simulink model "wasserpumpe"  (R2016b)
settings: Solver=VariableStepAuto  StartTime=0.0  StopTime=10  MaxStep=0.05  RelTol=1e-3  EnableMultiTasking=on
libraries: sh_lib x9, fl_lib x7, nesl_utility x4
CloseFcn:
  | try,close(h1_sh_well_jet_pump),end
  | clear h1_sh_well_jet_pump
  | 
  | 
  | clear simlog_sh_well_jet_pump
Description:
  | Well with Jet Pump
  | 
  | Copyright 2008-2016 The MathWorks, Inc.
settings Model: ExtModeAutoUpdateStatusClock=off  Creator=MathWorks  LastModifiedBy=user
settings DataIOCC: LimitDataPoints=on  MaxDataPoints=10000  SaveFormat=Array  SignalLoggingSaveFormat=ModelDataLogs  SignalLoggingName=logsout_sh_well_jet_pump
settings OptimizationCC: ExpressionDepthLimit=2147483647  InitFltsAndDblsToZero=on  LifeSpan=inf
settings DebuggingCC: SaveWithParameterizedLinksMsg=none  UnderspecifiedInitializationDetection=Classic  MergeDetectMultiDrivingBlocksExec=none  SignalResolutionControl=TryResolveAllWithWarning  SolverPrmCheckMsg=warning  MultiTaskDSMMsg=warning  MultiTaskCondExecSysMsg=none  FcnCallInpInsideContextMsg=warning  AllowSymbolicDim=off  StateNameClashWarn=warning  SFUnexpectedBacktrackingDiag=warning  SFNoUnconditionalDefaultTransitionDiag=warning  SFExecutionAtInitializationDiag=none
settings HardwareCC: ProdBitPerPointer=32  ProdBitPerSizeT=32  ProdBitPerPtrDiffT=32  ProdLargestAtomicFloat=None  ProdIntDivRoundTo=Undefined  ProdEndianess=Unspecified  ProdWordSize=32  ProdHWDeviceType=32-bit Generic
settings ModelReferenceCC: PropagateSignalLabelsOutOfModel=off
settings GRTTargetCC: TargetFcnLib=ansi_tfl_tmw.mat  TargetLangStandard=C89/C90 (ANSI)  GeneratePreprocessorConditionals=Disable all  CombineOutputUpdateFcns=off  GRTInterface=on
settings ConfigComp: CovMetricSettings=dw  CovHtmlReporting=on  CovSaveCumulativeToWorkspaceVar=on  CovSaveSingleToWorkspaceVar=on  CovShowResultsExplorer=off  CovExternalEMLEnable=off
settings SimscapeCC: SimscapeLogType=all  SimscapeLogSimulationStatistics=on  SimscapeLogName=simlog_sh_well_jet_pump  SimscapeLogDataHistory=10000

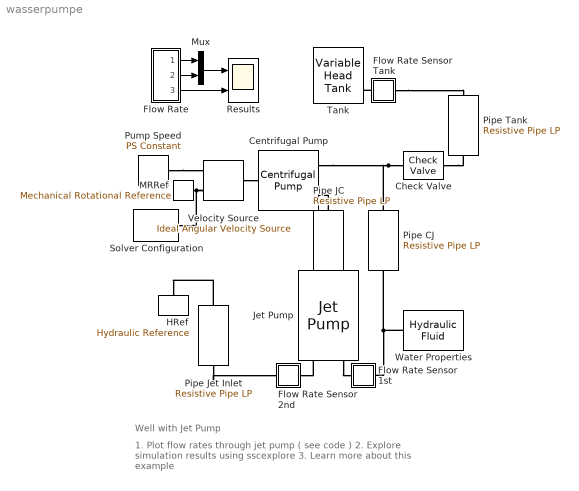
== system wasserpumpe ==
  note: Well with Jet Pump
  note: 1. Plot flow rates through jet pump ( see code )
      | 2. Explore simulation results using sscexplore
      | 3. Learn more about this example
  Centrifugal Pump : sh_lib/Pumps and Motors/Centrifugal Pump  mdl_type=2  c_1=326.8 Pa/(kg/m^3)  c_2=3.104e+4 Pa*s/kg  c_3=1.097e+7 Pa*s^2/(kg*m^3)  c_4=2.136e+5 Pa*s^2/(kg*m^3)  c_f=0.8  design_del=130 lpm  ref_velocity=1.77e+3 rpm  ref_density=940 kg/m^3  leak_resistance=1e+8 Pa/(m^3/s)  T_const=0.1 N*m  trq_press_coeff=1e-6 N*m/Pa  pump_del_1D="[ 0  0.076   0.24   0.35  0.416  0.492] m^3/s"  press_diff_1D=[3.514 3.246 2.6972 2.16 1.627 1.08] bar  pump_del_power_1D="[ 0  0.076   0.24   0.35  0.416  0.492] m^3/s"  power_1D="[0 0.58   1.57  1.79  1.61  1.27] kW"  pump_del_2D=[ 0 50 100 150 200 250 300 350 ] lpm  pump_vel_2D=[ 3.2e+3 3.3e+3 3.4e+3 3.5e+3 ] rpm  press_diff_2D=[ 8.3 8.8 9.3 9.9; 7.8 8.3 8.8 9.4; 7.2 7.6 8.2 8.7; 6.5 7 7.5 8; 5.6 6.1 6.6 7.1; 4.7 5.2 5.7 6.2; 3.4 4 4.4 4.9; 2.3 2.7 3.4 3.6 ] bar  pump_del_power_2D=[ 0 50 100 150 200 250 300 350 ] lpm  power_2D=[ 1.223e+3 1.341e+3 1.467e+3 1.6e+3; 1.414e+3 1.551e+3 1.696e+3 1.85e+3; 1.636e+3 1.794e+3 1.962e+3 2.14e+3; 1.941e+3 2.129e+3 2.326e+3 2.54e+3; 2.224e+3 2.439e+3 2.66e+3 2.91e+3; 2.453e+3 2.691e+3 2.947e+3 3.21e+3; 2.757e+3 3.024e+3 3.307e+3 3.608e+3; 2.945e+3 3.23e+3 3.533e+3 3.854e+3 ] W  interp_method=1  extrap_method=1
  Check Valve : sh_lib/Valves/Directional Valves/Check Valve  area_max=9.65 cm^2  pres_crack=0.055 bar  pres_max=0.172 bar  C_d=0.7  Re_cr=12  A_leak=1e-9 m^2  dynamic=0  tau=0.1 s  area_init=1e-12 m^2
  Flow Rate : Subsystem
  Flow Rate Sensor 1st : Subsystem
      mask Display: disp('Q1');
  Flow Rate Sensor 2nd : Subsystem
      mask Display: disp('Q2');
  Flow Rate Sensor Tank : Subsystem
      mask Display: disp('QT');
  HRef : fl_lib/Hydraulic/Hydraulic Elements/Hydraulic Reference
  Jet Pump : sh_lib/Pumps and Motors/Jet Pump  A_n=3 cm^2  A_th=6 cm^2  a=0.224  K_n=0.05  K_en=0.005  K_th=0.1  K_di=0.14
  MRRef : fl_lib/Mechanical/Rotational Elements/Mechanical Rotational Reference
  Mux : Mux  Inputs=2
  Pipe Jet Inlet : sh_lib/Low-Pressure Blocks/Resistive Pipe LP  cs_type=1  d_in=5 cm  area=1e-4 m^2  D_h=0.0112 m  s_factor=64  length=0.5 m  length_ad=1.5 m  roughness=1.5e-5 m  Re_lam=2e+3  Re_turb=4e+3  elevation_A=0 ft  elevation_B=-0.457 ft
  Pipe Tank : sh_lib/Low-Pressure Blocks/Resistive Pipe LP  cs_type=1  d_in=5 cm  area=1e-4 m^2  D_h=0.0112 m  s_factor=64  length=130 m  length_ad=15.5 m  roughness=1.5e-5 m  Re_lam=2e+3  Re_turb=4e+3  elevation_A=11 m  elevation_B=16 m
  Pipe CJ : sh_lib/Low-Pressure Blocks/Resistive Pipe LP  cs_type=1  d_in=6.35 cm  area=1e-4 m^2  D_h=0.0112 m  s_factor=64  length=11.5 m  length_ad=1.5 m  roughness=1.5e-5 m  Re_lam=2e+3  Re_turb=4e+3  elevation_A=11 m  elevation_B=-0.4572 m
  Pipe JC : sh_lib/Low-Pressure Blocks/Resistive Pipe LP  cs_type=1  d_in=10 cm  area=1e-4 m^2  D_h=0.0112 m  s_factor=64  length=11 m  length_ad=1.5 m  roughness=1.5e-5 m  Re_lam=2e+3  Re_turb=4e+3  elevation_A=11 ft  elevation_B=0 ft
  Pump Speed : fl_lib/Physical Signals/Sources/PS Constant  constant=1800/60*2*pi
  Results : Scope  NumInputPorts=2
  Solver Configuration : nesl_utility/Solver Configuration  PhysicalDomain=network_engine_domain  SubClassName=solver  LeftPortType=input  RightPortType=generic  Accelerate=off  Tones=[]  Harmonics=[]  SimulateNoise=off  Profile=off  UseLocalSampling=off  EnableSwitchedLinearOptims=on  FrequencyDomain=off  UseCCode=off  RelTol=0.001  AbsTol=1e-06  MinStep=1e-09  ToWorkspace=off  RevertToSquareIcSolve=off  NumHomotopyIterations=100  PhasorMode=off  PhasorModeNumHarmonics=1  OverrideAbsTol=off  DoDC=off  ResidualTolerance=1e-9  UseLocalSolver=off  LocalSolverChoice=NE_BACKWARD_EULER_ADVANCER  LocalSolverSampleTime=.001  DoFixedCost=off  MaxNonlinIter=3  MaxModeIter=2  LinearAlgebra=Sparse  DelaysMemoryBudget=1024  AutomaticFiltering=on  FilteringTimeConstant=0.001
  Tank : sh_lib/Low-Pressure Blocks/Variable Head Tank  init_volume=80 l  press=0 Pa  level_spec=1  tank_area=50 cm^2  fluid_volume_tab=[ 0 0.0028 0.0065 0.0114 0.0176 0.0252 0.0344 0.0436 0.0512 0.0574 0.0623 0.066 0.0688 0.0707 0.072 0.0727 ] m^3  fluid_level_tab=[ 0 0.02 0.04 0.06 0.08 0.1 0.12 0.14 0.16 0.18 0.2 0.22 0.24 0.26 0.28 0.3 ] m  pipe_diam=7.6 cm  loss_coeff=1.2  interp_method=1  extrap_method=1
  Velocity Source : fl_lib/Mechanical/Mechanical Sources/Ideal Angular Velocity Source
  Water Properties : sh_lib/Hydraulic Utilities/Hydraulic Fluid  DataSource=1  SelFluid=24  SysTemp=8  TrapAir=0.005  ViscDerFactor=1  range_error=2
  wires:
  Mux/1 -> Results/1
  Flow Rate/1(Q2) -> Mux/1
  Flow Rate/2(QT) -> Mux/2
  Flow Rate/3(Q1) -> Results/2
  connections:
  Flow Rate Sensor 2nd/RConn1 -- Jet Pump/LConn2
  Pipe Jet Inlet/RConn1 -- Flow Rate Sensor 2nd/LConn1
  Pipe JC/LConn1 -- Centrifugal Pump/RConn2
  Velocity Source/LConn1 -- Centrifugal Pump/LConn1
  Flow Rate Sensor Tank/LConn1 -- Pipe Tank/RConn1
  Flow Rate Sensor Tank/RConn1 -- Tank/RConn2
  MRRef/LConn1 -- Solver Configuration/RConn1 -- Velocity Source/RConn2
  Pump Speed/RConn1 -- Velocity Source/RConn1
  Check Valve/RConn1 -- Pipe Tank/LConn1
  Check Valve/LConn1 -- Pipe CJ/LConn1 -- Centrifugal Pump/RConn1
  Pipe JC/RConn1 -- Jet Pump/RConn1
  Jet Pump/LConn1 -- Flow Rate Sensor 1st/RConn1
  Pipe Jet Inlet/LConn1 -- HRef/LConn1
  Water Properties/RConn1 -- Pipe CJ/RConn1 -- Flow Rate Sensor 1st/LConn1

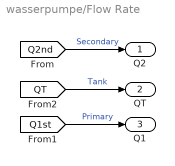
== system wasserpumpe/Flow Rate ==
  Q2 : Outport
  QT : Outport  Port=2
  Q1 : Outport  Port=3
  wires:
  [Q1st] -> Q1/1  "Primary"
  [Q2nd] -> Q2/1  "Secondary"
  [QT] -> QT/1  "Tank"

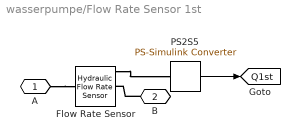
== system wasserpumpe/Flow Rate Sensor 1st ==
  Flow Rate Sensor : fl_lib/Hydraulic/Hydraulic Sensors/Hydraulic Flow Rate Sensor  Tag=Factory Generic
  PS2S5 : nesl_utility/PS-Simulink Converter  PhysicalDomain=network_engine_domain  SubClassName=ps_output  LeftPortType=input  RightPortType=output  PseudoPeriodic=off  Frequencies=[]  Unit=gpm  AffineConversion=off
  A : PMIOPort  Port=1  Side=Left
  B : PMIOPort  Port=2  Side=Right
  tag scope: Q1st=global
  wires:
  PS2S5/1 -> [Q1st]
  connections:
  B/RConn1 -- Flow Rate Sensor/RConn2
  A/RConn1 -- Flow Rate Sensor/LConn1
  Flow Rate Sensor/RConn1 -- PS2S5/LConn1

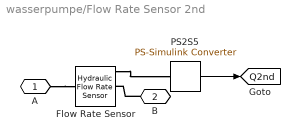
== system wasserpumpe/Flow Rate Sensor 2nd ==
  Flow Rate Sensor : fl_lib/Hydraulic/Hydraulic Sensors/Hydraulic Flow Rate Sensor  Tag=Factory Generic
  PS2S5 : nesl_utility/PS-Simulink Converter  PhysicalDomain=network_engine_domain  SubClassName=ps_output  LeftPortType=input  RightPortType=output  PseudoPeriodic=off  Frequencies=[]  Unit=gpm  AffineConversion=off
  A : PMIOPort  Port=1  Side=Left
  B : PMIOPort  Port=2  Side=Right
  tag scope: Q2nd=global
  wires:
  PS2S5/1 -> [Q2nd]
  connections:
  Flow Rate Sensor/RConn1 -- PS2S5/LConn1
  A/RConn1 -- Flow Rate Sensor/LConn1
  B/RConn1 -- Flow Rate Sensor/RConn2

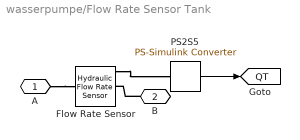
== system wasserpumpe/Flow Rate Sensor Tank ==
  Flow Rate Sensor : fl_lib/Hydraulic/Hydraulic Sensors/Hydraulic Flow Rate Sensor  Tag=Factory Generic
  PS2S5 : nesl_utility/PS-Simulink Converter  PhysicalDomain=network_engine_domain  SubClassName=ps_output  LeftPortType=input  RightPortType=output  PseudoPeriodic=off  Frequencies=[]  Unit=gpm  AffineConversion=off
  A : PMIOPort  Port=1  Side=Left
  B : PMIOPort  Port=2  Side=Right
  tag scope: QT=global
  wires:
  PS2S5/1 -> [QT]
  connections:
  Flow Rate Sensor/RConn1 -- PS2S5/LConn1
  A/RConn1 -- Flow Rate Sensor/LConn1
  B/RConn1 -- Flow Rate Sensor/RConn2
